simulink model "MPC_Kalman_Filter"  (R2022a)
settings: Solver=VariableStepAuto  StartTime=0.0  StopTime=10.0  RelTol=1e-3
values from neighbouring files (symbols this model uses):
  condDiscMat = BuildCondendsedMPCmatrices(discreteMat,r_Kalman,q_Kalman,F,f,PH)    [MAIN_MIMO.m]    (also in backupMain.m = BuildCondendsedMPCmatrices(discreteMat,r,q,F,f,PH); test.m = BuildCondendsedMPCmatrices(discreteMat,r,q,F,f,PH))
  discreteModel = c2d(continuousModel, info.Ts)    [MAIN_MIMO.m]    (also in backupMain.m; nonLinearPatient_main.m; test.m)
  PH = 200    [MAIN_MIMO.m]    (also in backupMain.m; nonLinearPatient_main.m; test.m)
  r = 0.01*eye(2)    [MAIN_MIMO.m]    (also in backupMain.m; nonLinearPatient_main.m; test.m)
undefined symbols (not defined in the file or in its folder): Discrete, info, myMPC_dist, op, Time
libraries: ctrlSharedLib x1
settings Model: Creator=user  LastModifiedBy=user

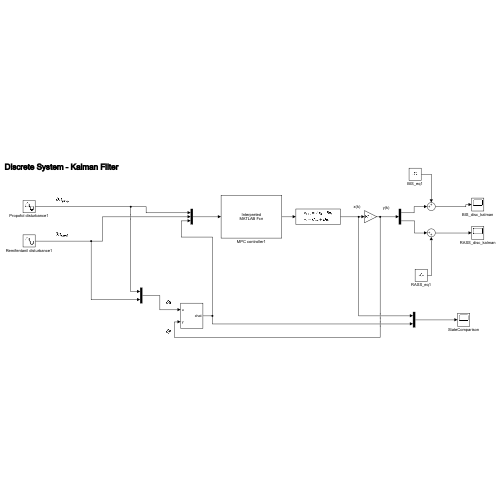
[thumbnail: Simulink's stored preview of the top-level diagram]
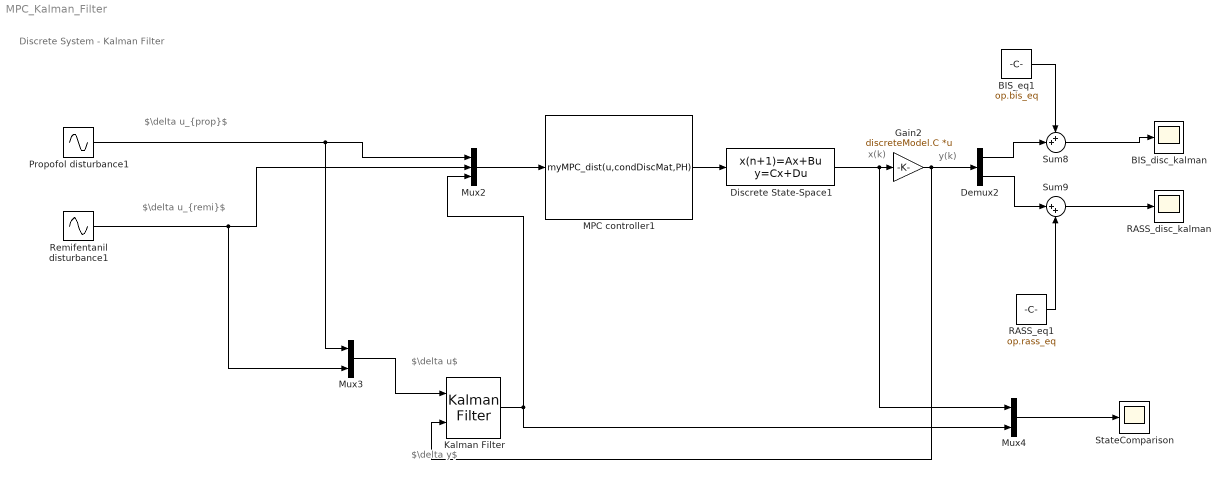
== system MPC_Kalman_Filter ==
  note: $\delta u$
  note: $\delta y$
  note: $\delta u_{remi}$
  note: $\delta u_{prop}$
  note: y(k)
  note: x(k)
  note: Discrete System - Kalman Filter
  BIS_disc_kalman : Scope
  BIS_eq1 : Constant  Value=op.bis_eq
  Demux2 : Demux  Outputs=2
  Discrete State-Space1 : DiscreteStateSpace  A=discreteModel.A  B=discreteModel.B  C=eye(size(discreteModel.A))  D=zeros(size(discreteModel.A,1),size(discreteModel.B,2))  SampleTime=info.Ts
  Gain2 : Gain  Gain=discreteModel.C  Multiplication=Matrix(K*u)
  Kalman Filter : ctrlSharedLib/Kalman Filter  TimeDomain=Discrete-Time  UseCurrentEstimator=on  ModelSource=LTI State-Space Variable  ModelSourceVariable=discreteModel  A=0.95  B=1  C=1  D=0  NumberOfStates=1  NumberOfInputs=1  NumberOfOutputs=1  InitialEstimateSource=Dialog  X0=0  P0=10  UseK=off  UseGH=off  NumberOfProcessNoiseInputs=1  G=1  TimeInvariantG=on  H=0  TimeInvariantH=on  Q=eye(10)  TimeInvariantQ=on  R=r  TimeInvariantR=on  N=0  TimeInvariantN=on  AddInputPort=on  AddEnablePort=off  OutputEstimatedY=off  OutputP=off  Ts=-1
  MPC controller1 : MATLABFcn  MATLABFcn=myMPC_dist(u,condDiscMat,PH)  OutputDimensions=2
  Mux2 : Mux  Inputs=3
  Mux3 : Mux  Inputs=2
  Mux4 : Mux  Inputs=2
  Propofol disturbance1 : Sin  Amplitude=0.3*op.propofol_eq  Frequency=1/500  SampleTime=info.Ts
  RASS_disc_kalman : Scope
  RASS_eq1 : Constant  Value=op.rass_eq
  Remifentanil disturbance1 : Sin  Amplitude=0.3*op.remifentanil_eq  Frequency=1/700  SampleTime=info.Ts
  StateComparison : Scope
  Sum8 : Sum  Inputs=++|
  Sum9 : Sum  Inputs=|++
  wires:
  Mux3/1 -> Kalman Filter/1
  Propofol disturbance1/1 -> Mux2/1, Mux3/1
  Sum8/1 -> BIS_disc_kalman/1
  Mux4/1 -> StateComparison/1
  Demux2/2 -> Sum9/1
  Remifentanil disturbance1/1 -> Mux3/2, Mux2/2
  Mux2/1 -> MPC controller1/1
  BIS_eq1/1 -> Sum8/1
  Discrete State-Space1/1 -> Mux4/1, Gain2/1
  Demux2/1 -> Sum8/2
  Gain2/1 -> Demux2/1, Kalman Filter/2
  RASS_eq1/1 -> Sum9/2
  MPC controller1/1 -> Discrete State-Space1/1
  Kalman Filter/1 -> Mux2/3, Mux4/2
  Sum9/1 -> RASS_disc_kalman/1
